simulink model "Mainframe"  (R2021a)
settings: Solver=FixedStepAuto  StartTime=0.0  StopTime=60  FixedStep=0.001  RelTol=1e-3
values from neighbouring files (symbols this model uses):
  den_lpf_d = den_lpf20    [Mainframe_init.m]    (also in load_autopilot.m)
  Emulated_FCC_IO_Delay = 7    [Mainframe_init.m]
  Enable_Gyros = 0    [Mainframe_init.m]
  Enable_INS = 0    [Mainframe_init.m]
  num_lpf_d = num_lpf20    [Mainframe_init.m]    (also in load_autopilot.m)
undefined symbols (not defined in the file or in its folder): act_dmp, act_omega, Actuator, Aerodynamics, aMode, Autopilot, AUX, c_b_WGS, c_be, c_flat, c_grav, c_h_geop0, c_h_geope, c_pa0, c_pe, c_r0, c_rot, c_rsma, c_Tmp0, d_siB_0, d_siB_max, d_siB_min, dd_siB_max, dd_siB_min, dev, DiscIntNeverNeededParam, e_pa, e_Tmp, fin_maxrate, flag_I_act_switch, flag_I_aero_switch, flag_I_flat, flag_I_gravity_switch, flag_I_rot, hcr, HIL_Data, JMMM_0, JMMM_e, JSPB_e, lat_0, lon_0, Mass_Props, mB_0, mM_0, mM_e, National_Instruments, Newton, pBII_0, PCIe, pMPB, pNPB, propellant_kg, prp_FBPB, prp_mdot, prp_T, pSPB, pwm_output1, qEG_0, qIB_0, qIE_0 ... (+31)
libraries: simulink_extras x38, simulink x31, custom_blocks x11, sldrtlib x10, aerolibcommonsys x4, px4Sensorslib x3, px4lib x3, aerolibnav x1
(part 1 of 17)
settings Model: SimulationMode=external  CodeVerificationMode=processor-in-the-loop (pil)  ExtModeTrigDuration=100000  Creator=m.hiepp  LastModifiedBy=corneto
settings SolverCC: AlgebraicLoopSolver=TrustRegion
settings DataIOCC: SignalLogging=off  ReturnWorkspaceOutputs=off
settings DebuggingCC: ParameterPrecisionLossMsg=none  SFMachineParentedDataDiag=warning  UnderSpecifiedDimensionMsg=warning  ArithmeticOperatorsInVariantConditions=warning
settings SFSimCC: CustomCodeUndefinedFunction=UseInterfaceOnly
settings RTWCC: Description=Simulink Desktop Real-Time  SystemTargetFile=sldrt.tlc  TemplateMakefile=sldrt.tmf  RTWCompilerOptimization=on
settings CodeAppCC: MaxIdLength=95
settings SimulinkDesktopRealTimeCC: TargetPreCompLibLocation=C:\Program Files\MATLAB\R2021a\toolbox\sldrt\lib\win64

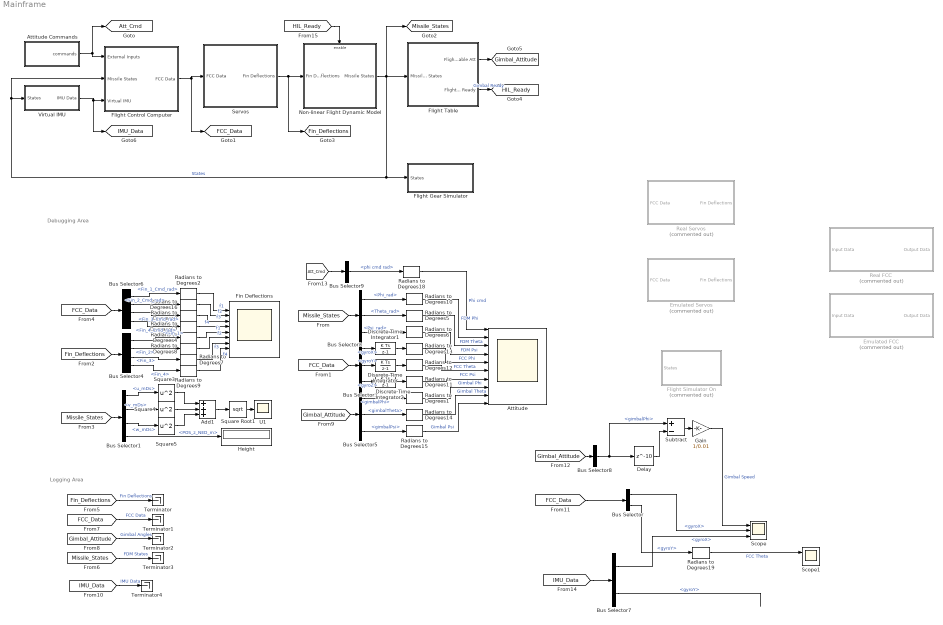
== system Mainframe ==
  note: Logging Area
  note: Debugging Area
  Add1 : Sum  Inputs=+++
  Attitude : Scope  NumInputPorts=10
  Attitude Commands : Subsystem
  Bus Selector : BusSelector  OutputSignals=Internal Data.gyroX,Internal Data.gyroY
  Bus Selector1 : BusSelector  OutputSignals=Translation_States.u_mDs,Translation_States.v_mDs,Translation_States.w_mDs,POS_NED.POS_z_NED_m
  Bus Selector2 : BusSelector  OutputSignals=Attitude_States.ATT_Euler.Phi_rad,Attitude_States.ATT_Euler.Theta_rad,Attitude_States.ATT_Euler.Psi_rad
  Bus Selector3 : BusSelector  OutputSignals=Internal Data.gyroX,Internal Data.gyroY,Internal Data.gyroZ
  Bus Selector4 : BusSelector  OutputSignals=Fin_1,Fin_2,Fin_3,Fin_4
  Bus Selector5 : BusSelector  OutputSignals=gimbalPhi,gimbalTheta,gimbalPsi
  Bus Selector6 : BusSelector  OutputSignals=Control Surface Cmd.Fin_1_Cmd_rad,Control Surface Cmd.Fin_2_Cmd_rad,Control Surface Cmd.Fin_3_Cmd_rad,Control Surface Cmd.Fin_4_Cmd_rad
  Bus Selector7 : BusSelector  OutputSignals=gyro.gyroX,gyro.gyroY
  Bus Selector8 : BusSelector  OutputSignals=gimbalPhi
  Bus Selector9 : BusSelector  OutputSignals=phi cmd rad
  Delay : Delay  DelayLength=10  SampleTime=0.001
  Discrete-Time Integrator : DiscreteIntegrator  SampleTime=0.01  ICPrevOutput=DiscIntNeverNeededParam  ICPrevScaledInput=DiscIntNeverNeededParam
  Discrete-Time Integrator1 : DiscreteIntegrator  SampleTime=0.01  ICPrevOutput=DiscIntNeverNeededParam  ICPrevScaledInput=DiscIntNeverNeededParam
  Discrete-Time Integrator2 : DiscreteIntegrator  SampleTime=0.01  ICPrevOutput=DiscIntNeverNeededParam  ICPrevScaledInput=DiscIntNeverNeededParam
  Emulated FCC : Subsystem  Commented=on  VariantControl=VSS_FCC_EMUL
  Emulated Servos : Subsystem  Commented=on  VariantControl=VSS_SERVOS_OFF
  Fin Deflections : Scope  NumInputPorts=8
  Flight Control Computer : Subsystem  VariantControl=VSS_FCC_REAL
  Flight Gear Simulator : Subsystem  Variant=on
  Flight Simulator On : Subsystem  Commented=on  VariantControl=VSS_FLIGHTGEAR_ON
  Flight Table : Subsystem  Variant=on
  Gain : Gain  Gain=1/0.01
  Height : Display
  Non-linear Flight Dynamic Model : Subsystem  VariantControl=VSS_FDM_SOPH
      mask init:
      | load('generated_FDM_params')
  Radians to Degrees{1..19} (19 alike) : simulink_extras/Transformations/Radians to Degrees
  Real FCC : Subsystem  Commented=on  VariantControl=VSS_FCC_REAL
  Real Servos : Subsystem  Commented=on  VariantControl=VSS_SERVOS_ON
  Scope : Scope  NumInputPorts=3
  Scope1 : Scope  NumInputPorts=2
  Servos : Subsystem  Variant=on
  Square Root1 : Sqrt  SaturateOnIntegerOverflow=on
  Square3 : Math  Operator=square  SaturateOnIntegerOverflow=on
  Square4 : Math  Operator=square  SaturateOnIntegerOverflow=on
  Square5 : Math  Operator=square  SaturateOnIntegerOverflow=on
  Subtract : Sum  Inputs=+-
  Terminator{,1..4} (5 alike) : Terminator
  U1 : Scope
  Virtual IMU : Subsystem
  tag scope: Att_Cmd=global, FCC_Data=global, Fin_Deflections=global, Gimbal_Attitude=global, HIL_Ready=global, IMU_Data=global, Missile_States=global
  wires:
  Bus Selector2/3 -> Radians to Degrees6/1  "<Psi_rad>"
  Bus Selector4/2 -> Radians to Degrees8/1  "<Fin_2>"
  Bus Selector2/2 -> Radians to Degrees5/1  "<Theta_rad>"
  Radians to Degrees9/1 -> Fin Deflections/8  "f4"
  Bus Selector3/3 -> Discrete-Time Integrator2/1  "<gyroZ>"
  Radians to Degrees7/1 -> Fin Deflections/7  "f3"
  [FCC_Data] -> Bus Selector3/1
  Radians to Degrees12/1 -> Attitude/6  "FCC Theta"
  Radians to Degrees15/1 -> Attitude/10  "Gimbal Psi"
  Radians to Degrees14/1 -> Attitude/9  "Gimbal Theta"
  Radians to Degrees8/1 -> Fin Deflections/6  "f2"
  Bus Selector2/1 -> Radians to Degrees10/1  "<Phi_rad>"
  Servos/1(Fin Deflections) -> [Fin_Deflections], Non-linear Flight Dynamic Model/1(Fin Deflections)
  Bus Selector4/1 -> Radians to Degrees4/1  "<Fin_1>"
  Bus Selector5/3 -> Radians to Degrees15/1  "<gimbalPsi>"
  [Fin_Deflections] -> Bus Selector4/1
  Radians to Degrees11/1 -> Attitude/7  "FCC Psi"
  Attitude Commands/1(commands) -> Flight Control Computer/1(External Inputs), [Att_Cmd]
  Bus Selector5/1 -> Radians to Degrees1/1  "<gimbalPhi>"
  Radians to Degrees1/1 -> Attitude/8  "Gimbal Phi"
  Radians to Degrees5/1 -> Attitude/3  "FDM Theta"
  Bus Selector5/2 -> Radians to Degrees14/1  "<gimbalTheta>"
  Flight Table/1(Flight Table Att) -> [Gimbal_Attitude]
  [Missile_States] -> Bus Selector2/1
  Non-linear Flight Dynamic Model/1(Missile States) -> Flight Control Computer/2(Missile States), Virtual IMU/1(States), Flight Gear Simulator/1(States), Flight Table/1(Missile States), [Missile_States]  "States"
  Bus Selector3/1 -> Discrete-Time Integrator1/1  "<gyroX>"
  Bus Selector4/3 -> Radians to Degrees7/1  "<Fin_3>"
  Radians to Degrees13/1 -> Attitude/5  "FCC Phi"
  Radians to Degrees4/1 -> Fin Deflections/5  "f1"
  Bus Selector3/2 -> Discrete-Time Integrator/1  "<gyroY>"
  Radians to Degrees10/1 -> Attitude/2  "FDM Phi"
  Bus Selector4/4 -> Radians to Degrees9/1  "<Fin_4>"
  Radians to Degrees6/1 -> Attitude/4  "FDM Psi"
  [Gimbal_Attitude] -> Bus Selector5/1
  Square Root1/1 -> U1/1
  Square4/1 -> Add1/2
  Square5/1 -> Add1/3
  Square3/1 -> Add1/1
  Add1/1 -> Square Root1/1
  Bus Selector1/3 -> Square5/1  "<w_mDs>"
  Bus Selector1/2 -> Square4/1  "<v_mDs>"
  Bus Selector1/1 -> Square3/1  "<u_mDs>"
  [Missile_States] -> Bus Selector1/1
  Bus Selector1/4 -> Height/1  "<POS_z_NED_m>"
  [FCC_Data] -> Bus Selector6/1
  Radians to Degrees2/1 -> Fin Deflections/1  "f1"
  Radians to Degrees16/1 -> Fin Deflections/2  "f2"
  Radians to Degrees3/1 -> Fin Deflections/3  "f3"
  Radians to Degrees17/1 -> Fin Deflections/4  "f4"
  Bus Selector6/1 -> Radians to Degrees2/1  "<Fin_1_Cmd_rad>"
  Bus Selector6/2 -> Radians to Degrees16/1  "<Fin_2_Cmd_rad>"
  Bus Selector6/3 -> Radians to Degrees3/1  "<Fin_3_Cmd_rad>"
  Bus Selector6/4 -> Radians to Degrees17/1  "<Fin_4_Cmd_rad>"
  [Fin_Deflections] -> Terminator/1  "Fin Deflections"
  [FCC_Data] -> Terminator1/1  "FCC Data"
  [Gimbal_Attitude] -> Terminator2/1  "Gimbal Angles"
  [Missile_States] -> Terminator3/1  "FDM States"
  Discrete-Time Integrator/1 -> Radians to Degrees12/1
  Discrete-Time Integrator1/1 -> Radians to Degrees13/1
  Discrete-Time Integrator2/1 -> Radians to Degrees11/1
  [IMU_Data] -> Bus Selector7/1
  Bus Selector7/1 -> Scope/3  "<gyroX>"
  [FCC_Data] -> Bus Selector/1
  Bus Selector/1 -> Scope/2  "<gyroX>"
  Bus Selector8/1 -> Subtract/1, Delay/1  "<gimbalPhi>"
  Delay/1 -> Subtract/2
  Subtract/1 -> Gain/1
  Gain/1 -> Scope/1  "Gimbal Speed"
  [Gimbal_Attitude] -> Bus Selector8/1
  [Att_Cmd] -> Bus Selector9/1
  Bus Selector9/1 -> Radians to Degrees18/1  "<phi cmd rad>"
  Radians to Degrees18/1 -> Attitude/1  "Phi cmd"
  Flight Control Computer/1(FCC Data) -> Servos/1(FCC Data), [FCC_Data]
  Flight Table/2(Flight Table Ready) -> [HIL_Ready]  "Gimbal Ready"
  Virtual IMU/1(" IMU Data") -> [IMU_Data], Flight Control Computer/3(Virtual IMU)
  Bus Selector/2 -> Radians to Degrees19/1  "<gyroY>"
  Bus Selector7/2 -> ?  "<gyroY>"
  Radians to Degrees19/1 -> Scope1/1  "FCC Theta"
  [IMU_Data] -> Terminator4/1  "IMU Data"
  [HIL_Ready] -> Non-linear Flight Dynamic Model/Enable

== system Mainframe/Attitude Commands ==
  Bus Creator : BusCreator  Inputs=3
  Delayed Sine : custom_blocks/Delayed Sine  amp=deg2rad(65)  bias=0  freq=pi/3  phase=0  onTime=5  duration=3
  Enabled Subsystem1 : Subsystem  TreatAsAtomicUnit=on
  Radians to Degrees : simulink_extras/Transformations/Radians to Degrees
  Scope : Scope
  Zero : Constant  Value=0  OutDataTypeStr=Inherit: Inherit via back propagation
  Zero1 : Constant  Value=0  OutDataTypeStr=Inherit: Inherit via back propagation
  commands : Outport
  wires:
  Delayed Sine/1 -> Radians to Degrees/1, Bus Creator/1  "phi cmd rad"
  Bus Creator/1 -> commands/1
  Zero/1 -> Bus Creator/3  "psi cmd rad"
  Zero1/1 -> Bus Creator/2  "theta cmd rad"
  Enabled Subsystem1/1(CalibrationTime) -> Delayed Sine/1  "Calibration Time"
  [HIL_Ready] -> Enabled Subsystem1/Trigger
  Radians to Degrees/1 -> Scope/1

== system Mainframe/Emulated FCC ==
  Input Data : Inport
  100 Hz : DiscretePulseGenerator  PulseType=Time based  Period=0.01  PulseWidth=50
  Delay : Delay  DelayLength=Emulated_FCC_IO_Delay  SampleTime=0.001
  Delay1 : Delay  DelayLength=Emulated_FCC_IO_Delay  SampleTime=0.001
  Emulated Pixhawk : Subsystem
  Output Data : Outport
  wires:
  Emulated Pixhawk/1(Serial Out) -> Delay1/1
  Input Data/1 -> Delay/1
  Delay1/1 -> Output Data/1
  Delay/1 -> Emulated Pixhawk/1(Serial In)
  100 Hz/1 -> Emulated Pixhawk/Trigger

== system Mainframe/Emulated Servos ==
  FCC Data : Inport
  Bus Creator : BusCreator  Inputs=4
  Bus Selector : BusSelector  OutputSignals=Control Surface Cmd.Fin_1_Cmd_rad,Control Surface Cmd.Fin_2_Cmd_rad,Control Surface Cmd.Fin_3_Cmd_rad,Control Surface Cmd.Fin_4_Cmd_rad
  Transfer Fcn{1..4} (4 alike) : TransferFcn  Numerator=33770  Denominator=[1 395.7 33770]
  Fin Deflections : Outport
  wires:
  FCC Data/1 -> Bus Selector/1
  Bus Selector/1 -> Transfer Fcn1/1  "<Fin_1_Cmd_rad>"
  Bus Selector/2 -> Transfer Fcn2/1  "<Fin_2_Cmd_rad>"
  Bus Selector/3 -> Transfer Fcn3/1  "<Fin_3_Cmd_rad>"
  Bus Selector/4 -> Transfer Fcn4/1  "<Fin_4_Cmd_rad>"
  Bus Creator/1 -> Fin Deflections/1
  Transfer Fcn1/1 -> Bus Creator/1  "Fin_1"
  Transfer Fcn2/1 -> Bus Creator/2  "Fin_2"
  Transfer Fcn3/1 -> Bus Creator/3  "Fin_3"
  Transfer Fcn4/1 -> Bus Creator/4  "Fin_4"

== system Mainframe/Flight Control Computer ==
  External Inputs : Inport
  Missile States : Inport  Port=2
  Virtual IMU : Inport  Port=3
  Bus Creator : BusCreator  Inputs=2
  Constant1 : Constant  Value=Enable_Gyros  OutDataTypeStr=single
  Constant4 : Constant  Value=Enable_INS  OutDataTypeStr=single
  Debug : Scope
  FCC - Real or Emulated : Subsystem  Variant=on
  FCC Sync : Scope
  Heartbeat Check : Subsystem
  In Sync : Subsystem
  Recieve from FCC : Subsystem
  Scope1 : Scope
  Send to FCC : Subsystem
  FCC Data : Outport
  wires:
  Constant4/1 -> Send to FCC/1(Enable INS Flag)
  Recieve from FCC/2(internal data) -> Bus Creator/2  "Internal Data"
  Recieve from FCC/1(fin_cmd_rad) -> Bus Creator/1  "Control Surface Cmd"
  External Inputs/1 -> Send to FCC/5(External Inputs)
  Missile States/1 -> Send to FCC/3(Missile States)
  Send to FCC/1(data out) -> FCC - Real or Emulated/1(Input Data)
  FCC - Real or Emulated/1(Output Data) -> Recieve from FCC/1(data in)
  Recieve from FCC/3(Other) -> Debug/1
  Constant1/1 -> Send to FCC/2(Enable Gyros Flag)
  Heartbeat Check/1(Communication Delay) -> Scope1/1
  Bus Creator/1 -> FCC Data/1  "FCC data"
  Virtual IMU/1 -> Send to FCC/4(Virtual IMU)
  In Sync/1(Heartbeat Sync) -> FCC Sync/1
  Send to FCC/2(Heartbeat Send) -> In Sync/1(send)
  Recieve from FCC/4(Output) -> In Sync/2(receive)

== system Mainframe/Flight Gear Simulator ==
  States : Inport
  Flight Simulator Off : Subsystem  VariantControl=VSS_FLIGHTGEAR_OFF
  Flight Simulator On : Subsystem  VariantControl=VSS_FLIGHTGEAR_ON

== system Mainframe/Flight Simulator On ==
  States : Inport
  Bus Selector1 : BusSelector  OutputSignals=POS_NED.POS_x_NED_m,POS_NED.POS_y_NED_m,POS_NED.POS_z_NED_m,Attitude_States.ATT_Euler.Phi_rad,Attitude_States.ATT_Euler.Theta_rad,Attitude_States.ATT_Euler.Psi_rad
  Demux : Demux  Outputs=2
  Flat Earth to LLA : Subsystem  mask(Flat Earth to LLA){units=Metric (MKS), ptype=Earth (WGS84), F=1/298.257223563, R=6378137, LL0=[32.086241 34.768375], psi=0}
      mask prompts: units "aeroblks:aeroblktransform:blockFlatEarthtoLLAParamUnits"; ptype "aeroblks:aeroblktransform:blockFlatEarthtoLLAParamPlanetmodel"; F "aeroblks:aeroblktransform:blockFlatEarthtoLLAParamFlattening"; R "aeroblks:aeroblktransform:blockFlatEarthtoLLAParamEquatorialradiusofplanet"; LL0 "aeroblks:aeroblktransform:blockFlatEarthtoLLAParamInitialgeodeticlatitudeandlongitudedeg"; psi "aeroblks:aeroblktransform:blockFlatEarthtoLLAParamDirectionofflatEarthxaxisdegreesclockwisefromnorth"
      mask help: aeroblks:aeroblktransform:blockFlatEarthtoLLADesc
      mask init:
      | aeroicon('aeroblklla')
      mask Help: eval('asbhelp');
      mask TypeOptions units: aeroblks:aeroblktransform:blockFlatEarthtoLLAParamComboMetricMKS | aeroblks:aeroblktransform:blockFlatEarthtoLLAParamComboEnglish
      mask TypeOptions ptype: aeroblks:aeroblktransform:blockFlatEarthtoLLAParamComboCustom | aeroblks:aeroblktransform:blockFlatEarthtoLLAParamComboEarthWGS84
      mask Callback ptype: aeroicon('aeroblklla')
      mask Display:
      | port_label('input',1,'X_{e}','texmode','on')
      | port_label('input',2,'h_{ref}','texmode','on')
      | port_label('output',1,'\mu l','texmode','on')
      | port_label('output',2,'h','texmode','on')
  FlightGear Preconfigured 6DoF Animation : Subsystem  TreatAsAtomicUnit=on  SimViewingDevice=on  mask(FlightGearQuick6DoFAnimation){xFlightGearVersion=v2018.3, DestinationIpAddress=127.0.0.1, DestinationPort=5502, SampleTime=0.001, packetVersion=24}
      mask prompts: xFlightGearVersion "aeroblks:aeroblkfltsims:blockFlightGearQuick6DoFAnimationParamFlightGearversion"; DestinationIpAddress "aeroblks:aeroblkfltsims:blockFlightGearQuick6DoFAnimationParamDestinationIPaddress"; DestinationPort "aeroblks:aeroblkfltsims:blockFlightGearQuick6DoFAnimationParamDestinationport"; SampleTime "aeroblks:aeroblkfltsims:blockFlightGearQuick6DoFAnimationParamSampletime1forinherited"; packetVersion "aeroblks:aeroblkfltsims:blockFlightGearPackNetParamFlightGearPacketversion"
      mask help: aeroblks:aeroblkfltsims:blockFlightGearQuick6DoFAnimationDesc
      mask init:
      | aeroicon('aeroblkfgsend');
      settings: AttributesFormatString=Version Selected: %<xFlightGearVersion>
      mask Help: eval('asbhelp(''flightgear_preconfigured_6dof_animation'')');
      mask TypeOptions xFlightGearVersion: aeroblks:aeroblkfltsims:blockFlightGearVersionCombov20 | aeroblks:aeroblkfltsims:blockFlightGearVersionCombov24 | aeroblks:aeroblkfltsims:blockFlightGearVersionCombov26 | aeroblks:aeroblkfltsims:blockFlightGearVersionCombov28 | aeroblks:aeroblkfltsims:blockFlightGearVersionCombov210 | aeroblks:aeroblkfltsims:blockFlightGearVersionCombov212 | aeroblks:aeroblkfltsims:blockFlightGearVersionCombov30 | aeroblks:aeroblkfltsims:blockFlightGearVersionCombov32 | aeroblks:aeroblkfltsims:blockFlightGearVersionCombov34 | aeroblks:aeroblkfltsims:blockFlightGearVersionCombov20161 | aeroblks:aeroblkfltsims:blockFlightGearVersionCombov20163 | aeroblks:aeroblkfltsims:blockFlightGearVersionCombov20171 | aeroblks:aeroblkfltsims:blockFlightGearVersionCombov20173 | aeroblks:aeroblkfltsims:blockFlightGearVersionCombov20181 | aeroblks:aeroblkfltsims:blockFlightGearVersionCombov20182 | aeroblks:aeroblkfltsims:blockFlightGearVersionCombov20183
      mask TypeOptions packetVersion: aeroblks:aeroblkfltsims:blockFlightGearPacketVersionCombo24
      mask DialogControl xFlightGearVersion Prompt: FlightGear version:
      mask DialogControl DestinationIpAddress Prompt: Destination IP address:
      mask DialogControl DestinationPort Prompt: Destination port:
      mask DialogControl SampleTime Prompt: Sample time (-1 for inherited):
      mask DialogControl packetVersion Prompt: FlightGear packet version:
      mask Display: port_label('input',1,'l,\mu,h,\phi,\theta,\psi','texmode','on')
  FlightGear1 : Subsystem  mask(FlightGear){}
      mask DialogControl Control2 Prompt: Please ensure you have FlightGear installed before proceeding
      mask DialogControl Control4 Prompt: Once FlightGear has finished loading you may minimize the terminal window and run the simulation
      mask DialogControl Control6 Prompt: Please note this feature is only supported in "normal mode"
      mask DialogControl Control5 Prompt: Launch
      mask DialogControl Control5 Callback:
      | simPath = which(bdroot);
      | idx = strfind(simPath,'\');
      | dirPath = simPath(1:idx(end));
      | LaunchFGPath = append(dirPath,'req\runfg.bat&');
      | system(LaunchFGPath)
      mask Display: disp("Launch\n FlightGear Simulator")
  Mux2 : Mux  Inputs=6
  Vector Concatenate : Concatenate  NumInputs=3
  Zero2 : Constant  Value=-10  OutDataTypeStr=Inherit: Inherit via back propagation
  wires:
  Vector Concatenate/1 -> Flat Earth to LLA/1(Xe)
  Flat Earth to LLA/1(mu l) -> Demux/1
  Demux/1 -> Mux2/2
  Zero2/1 -> Flat Earth to LLA/2(ground height)
  Mux2/1 -> FlightGear Preconfigured 6DoF Animation/1(In1)
  Bus Selector1/1 -> Vector Concatenate/1  "<POS_x_NED_m>"
  States/1 -> Bus Selector1/1
  Bus Selector1/2 -> Vector Concatenate/2  "<POS_y_NED_m>"
  Demux/2 -> Mux2/1
  Flat Earth to LLA/2(h) -> Mux2/3
  Bus Selector1/3 -> Vector Concatenate/3  "<POS_z_NED_m>"
  Bus Selector1/4 -> Mux2/4  "<Phi_rad>"
  Bus Selector1/6 -> Mux2/6  "<Psi_rad>"
  Bus Selector1/5 -> Mux2/5  "<Theta_rad>"

== system Mainframe/Flight Table ==
  Missile States : Inport
  Flight Table Off : Subsystem  VariantControl=VSS_GIMBAL_OFF
  Flight Table On : Subsystem  VariantControl=VSS_GIMBAL_ON
  Flight Table Att : Outport  InitialOutput=1
  Flight Table Ready : Outport  Port=2  InitialOutput=1

== system Mainframe/Non-linear Flight Dynamic Model ==
  Fin Deflections : Inport
  Enable : EnablePort
  Environment : Subsystem
  Extract States : Subsystem
  GRM_Airframe : Subsystem
      mask Display: image('$imagefile'); % Use "Edit Image" on toolstrip to change.
  Stop-Condition : Subsystem
  Subsystem1 : Subsystem  Commented=on
  Translate Fins : Subsystem
  Missile States : Outport  VectorParamsAs1DForOutWhenUnconnected=off
  wires:
  Fin Deflections/1 -> Translate Fins/1(Servo Deflections)
  Extract States/1(States) -> Missile States/1, Stop-Condition/1(States)  "States"
  Translate Fins/1(afinB) -> GRM_Airframe/1(siB_cmd)
  GRM_Airframe/1(airfr) -> Extract States/1(airfr_bus)
  Environment/1(env_glbl_bus) -> GRM_Airframe/2(T_sim_glbl)

== system Mainframe/Real FCC ==
  Input Data : Inport
  Enabled Subsystem : Subsystem  TreatAsAtomicUnit=on
  Extract Message : MATLAB Function  TreatAsAtomicUnit=on
  Packet Input : sldrtlib/Packet Input  SampleTime=0.001  MaxMissedTicks=10  ShowMissedTicks=off  YieldWhenWaiting=on  DrvName=Standard_Devices/Serial_Port  DrvAddress=3  DrvOptions=[115200 8 0 0 0 0 0 0]  PacketSize=FCC_message_size  DataTypes=FCC_types  ShowReady=on  ShowError=off  PacketID=1  ByteOrder=1  ShowTimestamp=off
      settings: AttributesFormatString=Serial Port [3]
  Packet Output : sldrtlib/Packet Output  SampleTime=0.01  MaxMissedTicks=10  ShowMissedTicks=off  YieldWhenWaiting=on  DrvName=Standard_Devices/Serial_Port  DrvAddress=3  DrvOptions=[115200 8 0 0 0 0 0 0]  PacketSize=23*4  DataTypes='23*single'  ShowReady=off  ShowError=off  PacketID=1  ByteOrder=1  InitialValue=[]  FinalValue=[]
      settings: AttributesFormatString=Serial Port [3]
  Terminator1 : Terminator
  Output Data : Outport
  wires:
  Input Data/1 -> Packet Output/1
  Packet Input/1 -> Enabled Subsystem/1(Hold)
  Enabled Subsystem/1(Pass) -> Extract Message/1(packet)
  Packet Input/2 -> Enabled Subsystem/Trigger
  Extract Message/2(Extracted_Data) -> Output Data/1
  Extract Message/1(Error_Msg) -> Terminator1/1

== system Mainframe/Real Servos ==
  FCC Data : Inport
  Bus Creator : BusCreator  Inputs=4
  Demux : Demux
  Encoder Input : sldrtlib/Encoder Input  SampleTime=0.001  MaxMissedTicks=10  ShowMissedTicks=off  YieldWhenWaiting=off  DrvName=National_Instruments/PCIe-6321  DrvAddress=4294967295  DrvOptions=[0 0 0 2 2 2 2]  Channels=1:4  QuadMode=3  IndexPulse=1  InputFilter=Inf  DataType=1
      settings: AttributesFormatString=National Instruments\nPCIe-6321 [auto]
  Reset Encoders : Subsystem
  Terminator : Terminator
  Ticks to rads : Gain  Gain=2*pi/4096
  Fin Deflections : Outport
  wires:
  Encoder Input/1 -> Ticks to rads/1
  FCC Data/1 -> Terminator/1
  Bus Creator/1 -> Fin Deflections/1
  Demux/3 -> Bus Creator/3  "Fin_3"
  Demux/2 -> Bus Creator/2  "Fin_2"
  Demux/1 -> Bus Creator/1  "Fin_1"
  Demux/4 -> Bus Creator/4  "Fin_4"
  [HIL_Ready] -> Reset Encoders/1(Reset Encoders)
  Ticks to rads/1 -> Reset Encoders/2(Encoder Readings)
  Reset Encoders/1(Fin Angles) -> Demux/1

== system Mainframe/Servos ==
  FCC Data : Inport
  Emulated Servos : Subsystem  VariantControl=VSS_SERVOS_OFF
  Real Servos : Subsystem  VariantControl=VSS_SERVOS_ON
  Fin Deflections : Outport

== system Mainframe/Virtual IMU ==
  States : Inport
  Bus Creator1 : BusCreator  Inputs=3
  Bus Creator10 : BusCreator  Inputs=2
  Bus Creator2 : BusCreator  Inputs=3
  Bus Selector : BusSelector  OutputSignals=Translation_States_Dot.u_dot_mDs2,Translation_States_Dot.v_dot_mDs2,Translation_States_Dot.w_dot_mDs2,Rotation_States.p_radDs,Rotation_States.q_radDs,Rotation_States.r_radDs,Rotation_States_Dot.p_dot_radDs2,Rotation_States_Dot.q_dot_radDs2,Rotation_States_Dot.r_dot_radDs2,Attitude_States.ATT_Euler.Phi_rad,Attitude_States.ATT_Euler.Theta_rad
  Constant1 : Constant  Value=[0,0,0]
  Demux8 : Demux  Outputs=3
  Demux9 : Demux  Outputs=3
  Gravity Vector : Subsystem
  Mux1 : Mux  Inputs=3
  Mux2 : Mux  Inputs=3
  Mux3 : Mux  Inputs=3
  Three-axis Inertial Measurement Unit : aerolibnav/Three-axis Inertial Measurement Unit  units=Metric (MKS)  imu=[0.43197 -0.00245 -0.01265]  i_Ts=0  dtype_a=on  w_a=190  z_a=0.707  a_sf_cc=[1.00135 0.0029375 0.00018125; -0.0029375 1.001525 0.0025625; -0.00018125 -0.0025625 1.004375]  a_bias=[0.086853 0.0258 -0.009194]  a_sat="[-156.921  -156.921  -156.921  156.921 156.921 156.921]"  dtype_g=on  w_g=190  z_g=0.707  g_sf_cc=[1.0045125 0.0045875 -0.005975; -0.0045875 1.0017125 0.0036875; 0.005975 -0.0036875 1.00243125]  g_bias=[-0.02167 0.011301 0.00202676]  g_sens=[0.000062068 0.0000443968 -0.0010608]  g_sat="[-34.9  -34.9  -34.9  34.9 34.9 34.9]"  i_rand=off  i_seeds=[23093 23094 23095 23096 23097 23098]  i_pow=[0.001 0.001 0.001 0.0001 0.0001 0.0001]
  " IMU Data" : Outport  VectorParamsAs1DForOutWhenUnconnected=off
  wires:
  Bus Selector/5 -> Mux2/2  "<q_radDs>"
  Mux3/1 -> Three-axis Inertial Measurement Unit/3
  Bus Selector/3 -> Mux1/3  "<w_dot_mDs2>"
  Bus Creator10/1 -> " IMU Data"/1  "Virtual IMU"
  Bus Selector/6 -> Mux2/3  "<r_radDs>"
  States/1 -> Bus Selector/1
  Bus Selector/11 -> Gravity Vector/2(Theta)  "<Theta_rad>"
  Bus Selector/2 -> Mux1/2  "<v_dot_mDs2>"
  Three-axis Inertial Measurement Unit/2 -> Demux9/1
  Bus Creator2/1 -> Bus Creator10/2  "gyro"
  Mux1/1 -> Three-axis Inertial Measurement Unit/1
  Mux2/1 -> Three-axis Inertial Measurement Unit/2
  Demux8/3 -> Bus Creator1/3  "accZ"
  Demux9/2 -> Bus Creator2/2  "gyroY"
  Demux9/1 -> Bus Creator2/1  "gyroX"
  Three-axis Inertial Measurement Unit/1 -> Demux8/1
  Demux8/1 -> Bus Creator1/1  "accX"
  Constant1/1 -> Three-axis Inertial Measurement Unit/4
  Bus Selector/4 -> Mux2/1  "<p_radDs>"
  Bus Creator1/1 -> Bus Creator10/1  "accelerometer"
  Demux8/2 -> Bus Creator1/2  "accY"
  Bus Selector/1 -> Mux1/1  "<u_dot_mDs2>"
  Gravity Vector/1(g) -> Three-axis Inertial Measurement Unit/5
  Demux9/3 -> Bus Creator2/3  "gyroZ"
  Bus Selector/10 -> Gravity Vector/1(Phi)  "<Phi_rad>"
  Bus Selector/8 -> Mux3/2  "<q_dot_radDs2>"
  Bus Selector/7 -> Mux3/1  "<p_dot_radDs2>"
  Bus Selector/9 -> Mux3/3  "<r_dot_radDs2>"

== system Mainframe/Attitude Commands/Enabled Subsystem1 ==
  Trigger : TriggerPort  VariantControl=Variant  PortDimensions=1
  Digital Clock : DigitalClock  SampleTime=-1
  CalibrationTime : Outport  InitialOutput=1e9
  wires:
  Digital Clock/1 -> CalibrationTime/1

== system Mainframe/Emulated FCC/Emulated Pixhawk ==
  Serial In : Inport
  Trigger : TriggerPort  VariantControl=Variant  PortDimensions=1
  Autopilot : Subsystem
  Convert to Bus : Subsystem
  Convert to Vector : Subsystem
  Fin Allocation : Subsystem
  Gyro : Subsystem
  IMU - Merge : Subsystem
  Inertial Navigation System : Subsystem
  Servo Commands : Subsystem
  Zero : Constant  Value=0  OutDataTypeStr=Inherit: Inherit via back propagation
  Serial Out : Outport
  tag scope: Heartbeat=global
  wires:
  [Real_Gyro_Data] -> Convert to Vector/4(Real Gyro Data)
  Convert to Bus/2(Ext. Commands) -> [Ext_Cmd]
  Autopilot/1(Attitude_Commands) -> Fin Allocation/1(Attitude Cmd)  "ATT_Cmd"
  Convert to Bus/3(Enable INS Flag) -> Inertial Navigation System/1(Enable INS Flag)
  Inertial Navigation System/1(INS Data) -> [INS_Data]
  Zero/1 -> Convert to Vector/5(Debug Port)
  [Ext_Cmd] -> Autopilot/1(Cmd)
  [Heartbeat] -> Convert to Vector/2(Heartbeat)
  [IMU_Data] -> Autopilot/2(IMU Data)
  [INS_Data] -> Autopilot/3(INS Data)
  Gyro/1(Real Gyro Data) -> [Real_Gyro_Data], IMU - Merge/3(Real Gyro)
  IMU - Merge/1(IMU Data) -> [IMU_Data], Inertial Navigation System/3(IMU Data)
  Convert to Vector/1(To HIL) -> Serial Out/1
  Fin Allocation/1(Fin Cmd) -> Servo Commands/1(Fin Cmd), Convert to Vector/1(Fin Deflections)
  Serial In/1 -> Convert to Bus/1(Input)
  [INS_Data] -> Convert to Vector/3(INS Data)
  Convert to Bus/5(Real Gyros Flag) -> IMU - Merge/1(Real Gyro Flag)
  Convert to Bus/4(Missile States) -> Inertial Navigation System/2(Missile States)
  Convert to Bus/1(Heartbeat) -> [Heartbeat]
  Convert to Bus/6(Virtual IMU Data) -> IMU - Merge/2(HIL IMU)

== system Mainframe/Flight Control Computer/FCC - Real or Emulated ==
  Input Data : Inport
  Emulated FCC : Subsystem  VariantControl=VSS_FCC_EMUL
  Real FCC : Subsystem  VariantControl=VSS_FCC_REAL
  Output Data : Outport

== system Mainframe/Flight Control Computer/Heartbeat Check ==
  note: This block ensures the Pixhawk is connected and functioning correctly
  Cast To Single : DataTypeConversion  OutDataTypeStr=single
  FCC Sync : Scope
  In Sync : Subsystem
  Mux : Mux  Inputs=2
  One : Constant  Value=9  OutDataTypeStr=Inherit: Inherit via back propagation
  Rate Transition : RateTransition  OutPortSampleTime=0.001
  Rate Transition1 : RateTransition  OutPortSampleTime=0.001
  Saturation : Saturate  UpperLimit=inf  LowerLimit=0
  Scope : Scope
  Subtract : Sum  Inputs=+--
  Communication Delay : Outport
  wires:
  [Heartbeat_Received] -> Rate Transition1/1  "receive"
  [Heartbeat_Sent] -> In Sync/1(send), Rate Transition/1
  Rate Transition/1 -> In Sync/2(receive), Subtract/1, Mux/1
  Rate Transition1/1 -> Subtract/2, Cast To Single/1
  Cast To Single/1 -> Mux/2
  Subtract/1 -> Saturation/1
  Saturation/1 -> Communication Delay/1  "FccDelay"
  One/1 -> Subtract/3
  Mux/1 -> Scope/1
  In Sync/1(Heartbeat Sync) -> FCC Sync/1

== system Mainframe/Flight Control Computer/In Sync ==
  note: This block ensures the Pixhawk is connected and functioning correctly
  send : Inport
  receive : Inport  Port=2
  Cast To Single : DataTypeConversion  OutDataTypeStr=single
  Mux : Mux  Inputs=2
  Rate Transition : RateTransition  OutPortSampleTime=0.001
  Rate Transition1 : RateTransition  OutPortSampleTime=0.001
  Heartbeat Sync : Outport
  wires:
  receive/1 -> Rate Transition1/1  "receive"
  send/1 -> Rate Transition/1
  Rate Transition/1 -> Mux/1
  Rate Transition1/1 -> Cast To Single/1
  Mux/1 -> Heartbeat Sync/1
  Cast To Single/1 -> Mux/2

== system Mainframe/Flight Control Computer/Recieve from FCC ==
  data in : Inport
  Bus Creator1 : BusCreator  Inputs=12
  Bus Creator4 : BusCreator  Inputs=4
  Cast To Double{,1..17} (18 alike) : DataTypeConversion  OutDataTypeStr=double
  Demux : Demux  Outputs=18
  Goto : Goto  Commented=on  GotoTag=Heartbeat_Received
  fin_cmd_rad : Outport  PortDimensions=4
  internal data : Outport  Port=2
  Other : Outport  Port=3
  Output : Outport  Port=4
  wires:
  data in/1 -> Demux/1
  Demux/1 -> Cast To Double/1
  Demux/7 -> Cast To Double6/1  "gyroY"
  Demux/11 -> Cast To Double10/1  "w"
  Demux/10 -> Cast To Double9/1  "v"
  Demux/9 -> Cast To Double8/1  "u"
  Demux/8 -> Cast To Double7/1  "gyroZ"
  Demux/4 -> Cast To Double3/1  "Fin_3_Cmd_rad"
  Demux/5 -> Cast To Double4/1  "Fin_4_Cmd_rad"
  Demux/3 -> Cast To Double2/1  "Fin_2_Cmd_rad"
  Demux/2 -> Cast To Double1/1  "Fin_1_Cmd_rad"
  Demux/6 -> Cast To Double5/1  "gyroX"
  Bus Creator4/1 -> fin_cmd_rad/1
  Bus Creator1/1 -> internal data/1
  Cast To Double/1 -> Output/1, Goto/1
  Cast To Double1/1 -> Bus Creator4/1  "Fin_1_Cmd_rad"
  Cast To Double2/1 -> Bus Creator4/2  "Fin_2_Cmd_rad"
  Cast To Double3/1 -> Bus Creator4/3  "Fin_3_Cmd_rad"
  Cast To Double4/1 -> Bus Creator4/4  "Fin_4_Cmd_rad"
  Cast To Double8/1 -> Bus Creator1/4  "u"
  Cast To Double9/1 -> Bus Creator1/5  "v"
  Cast To Double10/1 -> Bus Creator1/6  "w"
  Demux/12 -> Cast To Double12/1  "x"
  Demux/14 -> Cast To Double14/1  "z"
  Demux/15 -> Cast To Double15/1  "p"
  Demux/16 -> Cast To Double16/1  "q"
  Demux/17 -> Cast To Double11/1  "r"
  Demux/13 -> Cast To Double13/1  "y"
  Cast To Double12/1 -> Bus Creator1/7  "x"
  Cast To Double13/1 -> Bus Creator1/8  "y"
  Cast To Double14/1 -> Bus Creator1/9  "z"
  Demux/18 -> Cast To Double17/1
  Cast To Double17/1 -> Other/1  "debug"
  Cast To Double7/1 -> Bus Creator1/3  "gyroZ"
  Cast To Double6/1 -> Bus Creator1/2  "gyroY"
  Cast To Double5/1 -> Bus Creator1/1  "gyroX"
  Cast To Double15/1 -> Bus Creator1/10  "p"
  Cast To Double16/1 -> Bus Creator1/11  "q"
  Cast To Double11/1 -> Bus Creator1/12  "r"

== system Mainframe/Flight Control Computer/Send to FCC ==
  Enable INS Flag : Inport
  Enable Gyros Flag : Inport  Port=2
  Missile States : Inport  Port=3
  Virtual IMU : Inport  Port=4
  External Inputs : Inport  Port=5
  Bus Selector : BusSelector  OutputSignals=Translation_States.u_mDs,Translation_States.v_mDs,Translation_States.w_mDs,POS_NED.POS_x_NED_m,POS_NED.POS_y_NED_m,POS_NED.POS_z_NED_m,Rotation_States.p_radDs,Rotation_States.q_radDs,Rotation_States.r_radDs
  Bus Selector1 : BusSelector  OutputSignals=phi cmd rad
  Bus Selector2 : BusSelector  OutputSignals=accelerometer.accX,accelerometer.accY,accelerometer.accZ,gyro.gyroX,gyro.gyroY,gyro.gyroZ
  Bus Selector3 : BusSelector  OutputSignals=Attitude_States.ATT_Euler.Phi_rad,Attitude_States.ATT_Euler.Theta_rad,Attitude_States.ATT_Euler.Psi_rad
  Cast To Single{1..23} (23 alike) : DataTypeConversion  OutDataTypeStr=single
  Heartbeat Counter : Subsystem
  Mux : Mux  Inputs=23
  Scope : Scope
  data out : Outport
  Heartbeat Send : Outport  Port=2
  wires:
  Heartbeat Counter/1(Out1) -> Cast To Single18/1  "send"
  Enable INS Flag/1 -> Cast To Single17/1
  [HIL_Ready] -> Cast To Single19/1  "send"
  Mux/1 -> data out/1, Scope/1  "send"
  Missile States/1 -> Bus Selector3/1, Bus Selector/1
  Bus Selector1/1 -> Cast To Single20/1  "<phi cmd rad>"
  External Inputs/1 -> Bus Selector1/1
  Bus Selector/9 -> Cast To Single7/1  "<r_radDs>"
  Bus Selector2/1 -> Cast To Single6/1  "<accX>"
  Bus Selector2/2 -> Cast To Single5/1  "<accY>"
  Bus Selector2/3 -> Cast To Single4/1  "<accZ>"
  Bus Selector2/4 -> Cast To Single3/1  "<gyroX>"
  Bus Selector2/6 -> Cast To Single1/1  "<gyroZ>"
  Enable Gyros Flag/1 -> Cast To Single16/1
  Cast To Single1/1 -> Mux/19
  Bus Selector2/5 -> Cast To Single2/1  "<gyroY>"
  Cast To Single2/1 -> Mux/18
  Cast To Single3/1 -> Mux/17
  Cast To Single4/1 -> Mux/16
  Cast To Single5/1 -> Mux/15
  Cast To Single6/1 -> Mux/14
  Cast To Single7/1 -> Mux/13
  Cast To Single15/1 -> Mux/5
  Bus Selector/1 -> Cast To Single15/1  "<u_mDs>"
  Bus Selector/8 -> Cast To Single8/1  "<q_radDs>"
  Cast To Single8/1 -> Mux/12
  Cast To Single9/1 -> Mux/11
  Cast To Single10/1 -> Mux/10
  Cast To Single11/1 -> Mux/9
  Cast To Single12/1 -> Mux/8
  Cast To Single13/1 -> Mux/7
  Cast To Single14/1 -> Mux/6
  Bus Selector/2 -> Cast To Single14/1  "<v_mDs>"
  Bus Selector/3 -> Cast To Single13/1  "<w_mDs>"
  Bus Selector/4 -> Cast To Single12/1  "<POS_x_NED_m>"
  Bus Selector/5 -> Cast To Single11/1  "<POS_y_NED_m>"
  Bus Selector/6 -> Cast To Single10/1  "<POS_z_NED_m>"
  Bus Selector/7 -> Cast To Single9/1  "<p_radDs>"
  Cast To Single16/1 -> Mux/4
  Cast To Single17/1 -> Mux/3
  Cast To Single18/1 -> Heartbeat Send/1, [Heartbeat_Sent], Mux/2
  Cast To Single19/1 -> Mux/1
  Cast To Single20/1 -> Mux/23
  Bus Selector3/1 -> Cast To Single21/1  "<Phi_rad>"
  Cast To Single21/1 -> Mux/20
  Bus Selector3/3 -> Cast To Single23/1  "<Psi_rad>"
  Bus Selector3/2 -> Cast To Single22/1  "<Theta_rad>"
  Cast To Single22/1 -> Mux/21
  Cast To Single23/1 -> Mux/22
  Virtual IMU/1 -> Bus Selector2/1

== system Mainframe/Flight Gear Simulator/Flight Simulator Off ==
  States : Inport
  Terminator : Terminator
  wires:
  States/1 -> Terminator/1

== system Mainframe/Flight Gear Simulator/Flight Simulator On ==
  States : Inport
  Bus Selector1 : BusSelector  OutputSignals=POS_NED.POS_x_NED_m,POS_NED.POS_y_NED_m,POS_NED.POS_z_NED_m,Attitude_States.ATT_Euler.Phi_rad,Attitude_States.ATT_Euler.Theta_rad,Attitude_States.ATT_Euler.Psi_rad
  Demux : Demux  Outputs=2
  Flat Earth to LLA : Subsystem  mask(Flat Earth to LLA){units=Metric (MKS), ptype=Earth (WGS84), F=1/298.257223563, R=6378137, LL0=[32.086241 34.768375], psi=0}
      mask prompts: units "aeroblks:aeroblktransform:blockFlatEarthtoLLAParamUnits"; ptype "aeroblks:aeroblktransform:blockFlatEarthtoLLAParamPlanetmodel"; F "aeroblks:aeroblktransform:blockFlatEarthtoLLAParamFlattening"; R "aeroblks:aeroblktransform:blockFlatEarthtoLLAParamEquatorialradiusofplanet"; LL0 "aeroblks:aeroblktransform:blockFlatEarthtoLLAParamInitialgeodeticlatitudeandlongitudedeg"; psi "aeroblks:aeroblktransform:blockFlatEarthtoLLAParamDirectionofflatEarthxaxisdegreesclockwisefromnorth"
      mask help: aeroblks:aeroblktransform:blockFlatEarthtoLLADesc
      mask init:
      | aeroicon('aeroblklla')
      mask Help: eval('asbhelp');
      mask TypeOptions units: aeroblks:aeroblktransform:blockFlatEarthtoLLAParamComboMetricMKS | aeroblks:aeroblktransform:blockFlatEarthtoLLAParamComboEnglish
      mask TypeOptions ptype: aeroblks:aeroblktransform:blockFlatEarthtoLLAParamComboCustom | aeroblks:aeroblktransform:blockFlatEarthtoLLAParamComboEarthWGS84
      mask Callback ptype: aeroicon('aeroblklla')
      mask Display:
      | port_label('input',1,'X_{e}','texmode','on')
      | port_label('input',2,'h_{ref}','texmode','on')
      | port_label('output',1,'\mu l','texmode','on')
      | port_label('output',2,'h','texmode','on')
  FlightGear Preconfigured 6DoF Animation : Subsystem  TreatAsAtomicUnit=on  SimViewingDevice=on  mask(FlightGearQuick6DoFAnimation){xFlightGearVersion=v2018.3, DestinationIpAddress=127.0.0.1, DestinationPort=5502, SampleTime=0.001, packetVersion=24}
      mask prompts: xFlightGearVersion "aeroblks:aeroblkfltsims:blockFlightGearQuick6DoFAnimationParamFlightGearversion"; DestinationIpAddress "aeroblks:aeroblkfltsims:blockFlightGearQuick6DoFAnimationParamDestinationIPaddress"; DestinationPort "aeroblks:aeroblkfltsims:blockFlightGearQuick6DoFAnimationParamDestinationport"; SampleTime "aeroblks:aeroblkfltsims:blockFlightGearQuick6DoFAnimationParamSampletime1forinherited"; packetVersion "aeroblks:aeroblkfltsims:blockFlightGearPackNetParamFlightGearPacketversion"
      mask help: aeroblks:aeroblkfltsims:blockFlightGearQuick6DoFAnimationDesc
      mask init:
      | aeroicon('aeroblkfgsend');
      settings: AttributesFormatString=Version Selected: %<xFlightGearVersion>
      mask Help: eval('asbhelp(''flightgear_preconfigured_6dof_animation'')');
      mask TypeOptions xFlightGearVersion: aeroblks:aeroblkfltsims:blockFlightGearVersionCombov20 | aeroblks:aeroblkfltsims:blockFlightGearVersionCombov24 | aeroblks:aeroblkfltsims:blockFlightGearVersionCombov26 | aeroblks:aeroblkfltsims:blockFlightGearVersionCombov28 | aeroblks:aeroblkfltsims:blockFlightGearVersionCombov210 | aeroblks:aeroblkfltsims:blockFlightGearVersionCombov212 | aeroblks:aeroblkfltsims:blockFlightGearVersionCombov30 | aeroblks:aeroblkfltsims:blockFlightGearVersionCombov32 | aeroblks:aeroblkfltsims:blockFlightGearVersionCombov34 | aeroblks:aeroblkfltsims:blockFlightGearVersionCombov20161 | aeroblks:aeroblkfltsims:blockFlightGearVersionCombov20163 | aeroblks:aeroblkfltsims:blockFlightGearVersionCombov20171 | aeroblks:aeroblkfltsims:blockFlightGearVersionCombov20173 | aeroblks:aeroblkfltsims:blockFlightGearVersionCombov20181 | aeroblks:aeroblkfltsims:blockFlightGearVersionCombov20182 | aeroblks:aeroblkfltsims:blockFlightGearVersionCombov20183
      mask TypeOptions packetVersion: aeroblks:aeroblkfltsims:blockFlightGearPacketVersionCombo24
      mask DialogControl xFlightGearVersion Prompt: FlightGear version:
      mask DialogControl DestinationIpAddress Prompt: Destination IP address:
      mask DialogControl DestinationPort Prompt: Destination port:
      mask DialogControl SampleTime Prompt: Sample time (-1 for inherited):
      mask DialogControl packetVersion Prompt: FlightGear packet version:
      mask Display: port_label('input',1,'l,\mu,h,\phi,\theta,\psi','texmode','on')
  FlightGear1 : Subsystem  mask(FlightGear){}
      mask DialogControl Control2 Prompt: Please ensure you have FlightGear installed before proceeding
      mask DialogControl Control4 Prompt: Once FlightGear has finished loading you may minimize the terminal window and run the simulation
      mask DialogControl Control6 Prompt: Please note this feature is only supported in "normal mode"
      mask DialogControl Control5 Prompt: Launch
      mask DialogControl Control5 Callback:
      | simPath = which(bdroot);
      | idx = strfind(simPath,'\');
      | dirPath = simPath(1:idx(end));
      | LaunchFGPath = append(dirPath,'req\runfg.bat&');
      | system(LaunchFGPath)
      mask Display: disp("Launch\n FlightGear Simulator")
  Mux2 : Mux  Inputs=6
  Vector Concatenate : Concatenate  NumInputs=3
  Zero2 : Constant  Value=-10  OutDataTypeStr=Inherit: Inherit via back propagation
  wires:
  Vector Concatenate/1 -> Flat Earth to LLA/1(Xe)
  Flat Earth to LLA/1(mu l) -> Demux/1
  Demux/1 -> Mux2/2
  Zero2/1 -> Flat Earth to LLA/2(ground height)
  Mux2/1 -> FlightGear Preconfigured 6DoF Animation/1(In1)
  Bus Selector1/1 -> Vector Concatenate/1  "<POS_x_NED_m>"
  States/1 -> Bus Selector1/1
  Bus Selector1/2 -> Vector Concatenate/2  "<POS_y_NED_m>"
  Demux/2 -> Mux2/1
  Flat Earth to LLA/2(h) -> Mux2/3
  Bus Selector1/3 -> Vector Concatenate/3  "<POS_z_NED_m>"
  Bus Selector1/4 -> Mux2/4  "<Phi_rad>"
  Bus Selector1/6 -> Mux2/6  "<Psi_rad>"
  Bus Selector1/5 -> Mux2/5  "<Theta_rad>"

== system Mainframe/Flight Simulator On/Flat Earth to LLA ==
  Xe : Inport  Unit=m
  ground height : Inport  Port=2  Unit=m
  Disallow CGS : UnitConfiguration  UnitSystemsStr=English,SI,SI (extended)  AllowAllUnitSystems=off
  LatLong wrap : Subsystem
      mask init:
      | aeroicon('aeroblk')
      mask Display:
      | port_label('input',1,'[\mu l]','texmode','on')
      | port_label('output',1,'[\mu l]_{wrap}','texmode','on')
  LatLong wrap1 : Subsystem
      mask init:
      | aeroicon('aeroblk')
      mask Display:
      | port_label('input',1,'[\mu l]','texmode','on')
      | port_label('output',1,'[\mu l]_{wrap}','texmode','on')
  LongLat_offset : Subsystem
  Sel1 : Selector  InputPortWidth=3  IndexOptions=Index vector (dialog)  Indices=[1,2]  OutputSizes=1
  Sel2 : Selector  InputPortWidth=3  IndexOptions=Index vector (dialog)  Indices=3  OutputSizes=1
  Sum : Sum  Inputs=|++
  Sum1 : Sum  Inputs=-+
  "Xe " : InportShadow  Unit=m
  Ze2height : UnaryMinus
  initial_latg : Selector  InputPortWidth=2  IndexOptions=Index vector (dialog)  Indices=[1]  OutputSizes=1
  initial_pos : Constant  Value=LL0
  pos_deg : Subsystem
  mu l : Outport  Unit=deg  VectorParamsAs1DForOutWhenUnconnected=off
  h : Outport  Port=2  Unit=m  VectorParamsAs1DForOutWhenUnconnected=off
  wires:
  pos_deg/1(out) -> Sum/1
  LongLat_offset/1(DeltaLL_rad) -> pos_deg/1(in)
  LatLong wrap1/1(Lat/Long wrapped) -> initial_latg/1, Sum/2
  initial_pos/1 -> LatLong wrap1/1(LatLong)
  LatLong wrap/1(Lat/Long wrapped) -> mu l/1
  initial_latg/1 -> LongLat_offset/2(mu)
  "Xe "/1 -> Sel2/1
  Sel1/1 -> LongLat_offset/1(XY)
  ground height/1 -> Sum1/1
  Sum1/1 -> h/1
  Ze2height/1 -> Sum1/2  "alt"
  Sel2/1 -> Ze2height/1
  Sum/1 -> LatLong wrap/1(LatLong)
  Xe/1 -> Sel1/1

== system Mainframe/Flight Simulator On/FlightGear Preconfigured 6DoF Animation ==
  In1 : Inport
  Angle Conversion : Subsystem
  Angle Conversion1 : Subsystem
  Demux : Demux  Outputs=6
  Pack net_fdm Packet for FlightGear : S-Function  FunctionName=saerofgpacknetfdm  Parameters=packetVersion, 'on','off','off','off','off','off', SampleTime  SFunctionDeploymentMode=off  EnableBusSupport=off
  PacketSize : Constant  Value=408
  Rate Transition : RateTransition  Integrity=off  Deterministic=off  OutPortSampleTime=SampleTime
  Simulation Pace : S-Function  FunctionName=saeroclockpacer  Parameters=SimulationPace,SleepMode,OutputPaceError,SampleTime  SFunctionDeploymentMode=off  EnableBusSupport=off  mask(Simulation Pace){SimulationPace=1, SleepMode=MATLAB Thread, OutputPaceError=off, SampleTime=SampleTime}
      mask prompts: SimulationPace "aeroblks:aeroblkanimutils:blockSimulationPaceParamSimulationpacesimsecperclocksec"; SleepMode "aeroblks:aeroblkanimutils:blockSimulationPaceParamSleepmode"; OutputPaceError "aeroblks:aeroblkanimutils:blockSimulationPaceParamOutputpaceerrorsec"; SampleTime "aeroblks:aeroblkanimutils:blockSimulationPaceParamSampletime1forinherited"
      mask help: aeroblks:aeroblkanimutils:blockSimulationPaceDesc
      mask init:
      | aeroicon('aeroblkpacer');
      settings: AttributesFormatString=%<SimulationPace> sec/sec
      mask Help: eval('asbhelp');
      mask TypeOptions SleepMode: aeroblks:aeroblkanimutils:blockSimulationPaceParamComboOff | aeroblks:aeroblkanimutils:blockSimulationPaceParamComboMATLABThread | aeroblks:aeroblkanimutils:blockSimulationPaceParamComboBusyWait | aeroblks:aeroblkanimutils:blockSimulationPaceParamComboAuto
      mask DialogControl SimulationPace Prompt: Simulation pace (sim sec per clock sec):
      mask DialogControl SleepMode Prompt: Sleep mode:
      mask DialogControl OutputPaceError Prompt: Output pace error (sec)
      mask DialogControl SampleTime Prompt: Sample time (-1 for inherited):
      mask Display:
      | text(0.5,0.60,'Set','horizontalAlignment','center');
      | text(0.5,0.40,'Pace','horizontalAlignment','center');
  UDP Send : S-Function  FunctionName=saerofgsend  Parameters=DestinationIpAddress,DestinationPort,-1,SampleTime,0  SFunctionDeploymentMode=off  EnableBusSupport=off
  Unit Sys : UnitConfiguration  UnitSystemsStr=SI,SI (extended)  AllowAllUnitSystems=off
  toSingle1 : DataTypeConversion  OutDataTypeStr=single
  toSingle2 : DataTypeConversion  OutDataTypeStr=single
  toSingle3 : DataTypeConversion  OutDataTypeStr=single
  wires:
  Angle Conversion1/1(out) -> Pack net_fdm Packet for FlightGear/2
  Angle Conversion/1(out) -> Pack net_fdm Packet for FlightGear/1
  Rate Transition/1 -> Demux/1
  toSingle3/1 -> Pack net_fdm Packet for FlightGear/6
  toSingle2/1 -> Pack net_fdm Packet for FlightGear/5
  toSingle1/1 -> Pack net_fdm Packet for FlightGear/4
  Pack net_fdm Packet for FlightGear/1 -> UDP Send/1
  In1/1 -> Rate Transition/1
  Demux/1 -> Angle Conversion/1(in)
  Demux/2 -> Angle Conversion1/1(in)
  Demux/3 -> Pack net_fdm Packet for FlightGear/3
  Demux/4 -> toSingle1/1
  Demux/5 -> toSingle2/1
  Demux/6 -> toSingle3/1
  PacketSize/1 -> UDP Send/2

== system Mainframe/Flight Simulator On/FlightGear1 ==

== system Mainframe/Flight Table/Flight Table Off ==
  Missile States : Inport
  Bus Creator : BusCreator  Inputs=3
  Delay : Delay  DelayLength=1
  One : Constant  OutDataTypeStr=Inherit: Inherit via back propagation
  Terminator3 : Terminator
  Zero : Constant  Value=0  OutDataTypeStr=Inherit: Inherit via back propagation
  Zero1 : Constant  Value=0  OutDataTypeStr=Inherit: Inherit via back propagation
  Zero2 : Constant  Value=0  OutDataTypeStr=Inherit: Inherit via back propagation
  Flight Table Att : Outport  InitialOutput=1
  Flight Table Ready : Outport  Port=2  InitialOutput=1
  wires:
  Zero/1 -> Bus Creator/2  "gimbalTheta"
  Zero1/1 -> Bus Creator/1  "gimbalPhi"
  Zero2/1 -> Bus Creator/3  "gimbalPsi"
  One/1 -> Delay/1
  Missile States/1 -> Terminator3/1
  Bus Creator/1 -> Flight Table Att/1
  Delay/1 -> Flight Table Ready/1

== system Mainframe/Flight Table/Flight Table On ==
  Missile States : Inport
  Bus Creator : BusCreator  Inputs=3
  Bus Selector1 : BusSelector  OutputSignals=Attitude_States.ATT_Euler
  Configure Gimbals : Subsystem
  Current Attitude : Subsystem
  Stage 1 - Spin 360deg to find indexes : Subsystem
  "Stage 2 - Set gimbals to initial attitude " : Subsystem
  Stage 3 - Track Attitude Commands : Subsystem
  Flight Table Att : Outport  InitialOutput=1
  Flight Table Ready : Outport  Port=2  InitialOutput=1
  wires:
  Missile States/1 -> Bus Selector1/1
  Bus Creator/1 -> Flight Table Att/1
  [stage2complete] -> Flight Table Ready/1
  Current Attitude/1(gimbalPhi) -> Bus Creator/1
  Current Attitude/2(gimbalTheta) -> Bus Creator/2
  Current Attitude/3(gimbalPsi) -> Bus Creator/3
  Bus Selector1/1 -> Stage 3 - Track Attitude Commands/1(Attitude Cmd)  "<ATT_Euler>"

== system Mainframe/Non-linear Flight Dynamic Model/Environment ==
  Add : Sum  Inputs=-+
  Bus Creator1 : BusCreator  Inputs=5
  Clock : Clock
  Constant6 : Constant  Value=T_sim_lnch
  Enabled Subsystem1 : Subsystem  TreatAsAtomicUnit=on
  From10 : From  Commented=on  GotoTag=HIL_Ready  TagVisibility=global
  Memory : Memory
  NOT : Logic  Operator=NOT  IconShape=distinctive  AllPortsSameDT=off  OutDataTypeStr=boolean
  atm_dynamic : Subsystem
  deviation_Tmp : Constant  Value=e_Tmp
  deviation_pa_QFH : Constant  Value=e_pa
  env_glbl_bus : Outport
  wires:
  atm_dynamic/1(vWEG) -> Bus Creator1/3
  Bus Creator1/1 -> env_glbl_bus/1  "env_glbl_bus"
  Clock/1 -> Add/2
  Constant6/1 -> Bus Creator1/2  "T_sim_lnch"
  deviation_pa_QFH/1 -> Bus Creator1/5  "e_pa"
  deviation_Tmp/1 -> Bus Creator1/4  "e_Tmp"
  From10/1 -> ?
  Add/1 -> Bus Creator1/1  "T_sim_glbl"
  Enabled Subsystem1/1(CalibrationTime) -> Add/1, NOT/1
  Memory/1 -> Enabled Subsystem1/Enable
  NOT/1 -> Memory/1

== system Mainframe/Non-linear Flight Dynamic Model/Extract States ==
  airfr_bus : Inport
  Assemble_States_Bus1 : Subsystem
  Bus Selector1 : BusSelector  OutputSignals=flight_dyn_bus.vBIB,flight_dyn_bus.wBIB,flight_dyn_bus.aBIB,flight_dyn_bus.d_wBIB,flight_dyn_bus.qIB,flight_dyn_bus.pBII,flight_dyn_bus.vBII
  MATLAB Function1 : MATLAB Function  TreatAsAtomicUnit=on
  quaternion_to_euler_angles1 : Subsystem
      mask help: transforms quaternions to Euler angles (roll, pitch, yaw)
      mask Help:
      | Name:
      | 
      |     quaternion_to_euler_angles
      | 
      | Description:
      | 
      |     This block implements the transformation of a quaternion into the
      |     corresponding Euler angles (zyx-sequence, roll, pitch, yaw).
      | 
      | Inputs  [size] [data type] [unit]:
      | 
      |     quaternion  [4] [double] [-]
      | 
      | Outputs  [size] [data type] [unit]:
      | 
      |     roll angle phi  [1] [double] [rad]
      |     pitch angle theta  [1] [double] [rad]
      |     yaw angle psi  [1] [double] [rad]
      mask Display:
      | %disp (' q --> (Phi,Theta,Psi) [rad]')
      | disp('q \rightarrow eu(\Phi;\Theta;\Psi)','texmode','on')
  States : Outport
  wires:
  Bus Selector1/6 -> Assemble_States_Bus1/6(POS_NED)  "<pBII>"
  quaternion_to_euler_angles1/1(eulx) -> Assemble_States_Bus1/5(Attitude_States)  "from Quat"
  MATLAB Function1/1(q_conj) -> quaternion_to_euler_angles1/1(q)
  Bus Selector1/5 -> MATLAB Function1/1(q)  "<qIB>"
  airfr_bus/1 -> Bus Selector1/1
  Bus Selector1/1 -> Assemble_States_Bus1/1(Translation_States)  "<vBIB>"
  Bus Selector1/2 -> Assemble_States_Bus1/2(Rotation_States)  "<wBIB>"
  Bus Selector1/4 -> Assemble_States_Bus1/4(Rotation_States_Dot)  "<d_wBIB>"
  Bus Selector1/3 -> Assemble_States_Bus1/3(Translation_States_Dot)  "<aBIB>"
  Assemble_States_Bus1/1(States) -> States/1
  Bus Selector1/7 -> Assemble_States_Bus1/7(POS_NED_dot)  "<vBII>"
